simulink model "shabishiyan"  (R2021b)
settings: Solver=ode1  StartTime=0  StopTime=inf  FixedStep=0.005  RelTol=1e-3  EnableMultiTasking=on
libraries: gtbox x7, simulink x2
settings Model: SimulationMode=external  Creator=Administrator  LastModifiedBy=admin
settings SolverCC: AlgebraicLoopSolver=TrustRegion  AutoInsertRateTranBlk=on
settings DataIOCC: LimitDataPoints=on  SaveFormat=Array  ReturnWorkspaceOutputs=off
settings OptimizationCC: ExpressionDepthLimit=2147483647
settings DebuggingCC: UnderspecifiedInitializationDetection=Classic  MergeDetectMultiDrivingBlocksExec=none  SolverPrmCheckMsg=warning  MultiTaskRateTransMsg=warning  StateNameClashWarn=warning  SFUnexpectedBacktrackingDiag=warning  SFNoUnconditionalDefaultTransitionDiag=warning  SFExecutionAtInitializationDiag=none  SFMachineParentedDataDiag=warning  ArithmeticOperatorsInVariantConditions=warning
settings ModelReferenceCC: PropagateSignalLabelsOutOfModel=off
settings SFSimCC: SimUseLocalCustomCode=off  CustomCodeUndefinedFunction=UseInterfaceOnly
settings RTWCC: Description=Simulink Desktop Real-Time  SystemTargetFile=sldrt.tlc  TemplateMakefile=sldrt.tmf  RTWUseLocalCustomCode=off  RTWCompilerOptimization=on
settings CodeAppCC: MaxIdLength=95  StateflowObjectComments=on
settings SimulinkDesktopRealTimeCC: TargetPreCompLibLocation=C:\Program Files\MATLAB\R2021b\toolbox\sldrt\lib\win64  TargetLangStandard=C89/C90 (ANSI)  SupportVariableSizeSignals=off
settings ConfigComp: CovMetricSettings=dw  CovSaveCumulativeToWorkspaceVar=on  CovSaveSingleToWorkspaceVar=on  CovExternalEMLEnable=off

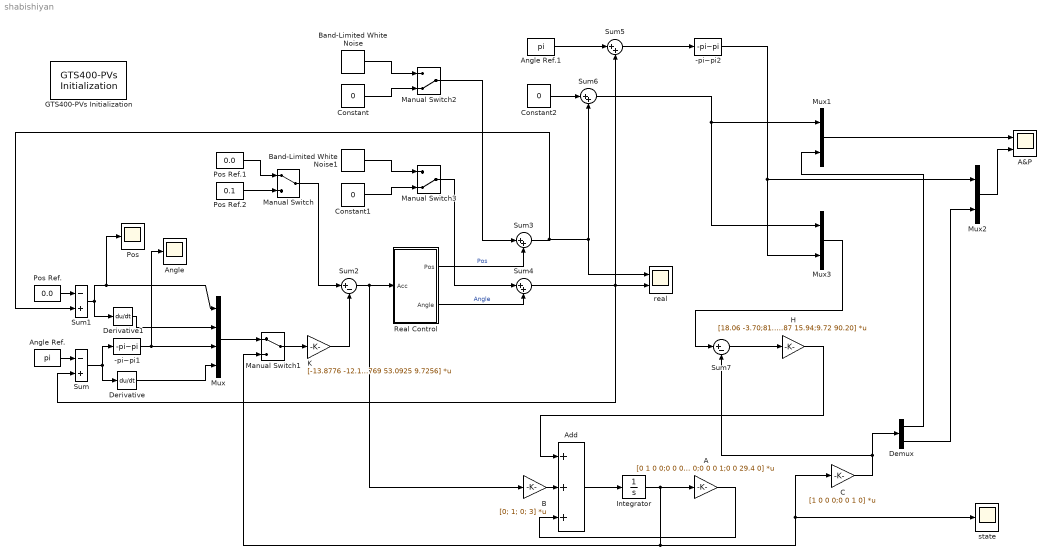
== system shabishiyan ==
  " -pi~pi1" : gtbox/GT-400-SV Function Blocks/ -pi~pi  Priority=1
      settings: SourceProductName=Googol Education Products v2.0
  " -pi~pi2" : gtbox/GT-400-SV Function Blocks/ -pi~pi  Priority=1
      settings: SourceProductName=Googol Education Products v2.0
  A : Gain  Gain=[0 1 0 0;0 0 0 0;0 0 0 1;0 0 29.4 0]  Multiplication=Matrix(K*u)
  A&P : Scope  NumInputPorts=2
  Add : Sum  Inputs=+++
  Angle : Scope
  Angle Ref. : Constant  Value=pi
  Angle Ref.1 : Constant  Value=pi
  B : Gain  Gain=[0; 1; 0; 3]  Multiplication=Matrix(K*u)
  Band-Limited White Noise : simulink/Sources/Band-Limited White Noise  Cov=[0.00001]  Ts=0.1  seed=[23341]
  Band-Limited White Noise1 : simulink/Sources/Band-Limited White Noise  Cov=[0.00001]  Ts=0.1  seed=[23341]
  C : Gain  Gain=[1 0 0 0;0 0 1 0]  Multiplication=Matrix(K*u)
  Constant : Constant  Value=0
  Constant1 : Constant  Value=0
  Constant2 : Constant  Value=0
  Demux : Demux  Outputs=2
  Derivative : Derivative
  Derivative1 : Derivative
  GTS400-PVs Initialization : gtbox/GTS-400-PV Function Blocks/GTS400-PVs Initialization  Priority=0  open=0  mode=0  servo=[1 0 0 0]  aft=[0 0 0 0]  pid1=[4.5 0 10]  pid2=[1 0 0]  pid3=[1 0 0]  pid4=[1 0 0]  enc1=on  enc2=on  enc3=on  enc4=on  lmt1=off  lmt2=off  lmt3=off  lmt4=off  cdno=1
      settings: SourceProductName=Googol Education Products v2.0
  H : Gain  Gain=[18.06 -3.70;81.37 -29.22;1.87 15.94;9.72 90.20]  Multiplication=Matrix(K*u)
  Integrator : Integrator
  K : Gain  Gain=[-13.8776 -12.1769 53.0925 9.7256]  Multiplication=Matrix(K*u)
  Manual Switch : ManualSwitch
  Manual Switch1 : ManualSwitch
  Manual Switch2 : ManualSwitch  CurrentSetting=0
  Manual Switch3 : ManualSwitch  CurrentSetting=0
  Mux : Mux
  Mux1 : Mux  Inputs=2
  Mux2 : Mux  Inputs=2
  Mux3 : Mux  Inputs=2
  Pos : Scope
  Pos Ref. : Constant  Value=0.0
  Pos Ref.1 : Constant  Value=0.0
  Pos Ref.2 : Constant  Value=0.1
  Real Control : Subsystem
  Sum : Sum  Inputs=-+  SaturateOnIntegerOverflow=on
  Sum1 : Sum  Inputs=-+  SaturateOnIntegerOverflow=on
  Sum2 : Sum  Inputs=|+-
  Sum{3..6} (4 alike) : Sum  Inputs=|++
  Sum7 : Sum  Inputs=|+-
  real : Scope  NumInputPorts=2
  state : Scope
  wires:
  Mux/1 -> Manual Switch1/1
  Sum/1 -> " -pi~pi1"/1, Derivative/1
  Derivative1/1 -> Mux/2
  Sum4/1 -> Sum5/2, real/2, Sum/2
  Derivative/1 -> Mux/4
  Sum3/1 -> real/1, Sum6/2, Sum1/2
  Pos Ref./1 -> Sum1/1
  Angle Ref./1 -> Sum/1
  " -pi~pi1"/1 -> Mux/3, Angle/1
  Sum1/1 -> Derivative1/1, Mux/1, Pos/1
  Pos Ref.1/1 -> Manual Switch/1
  Pos Ref.2/1 -> Manual Switch/2
  Manual Switch1/1 -> K/1
  Manual Switch/1 -> Sum2/1
  K/1 -> Sum2/2
  Band-Limited White Noise/1 -> Manual Switch2/1
  Constant/1 -> Manual Switch2/2
  Constant1/1 -> Manual Switch3/2
  Band-Limited White Noise1/1 -> Manual Switch3/1
  Manual Switch2/1 -> Sum3/1
  Real Control/1(Pos) -> Sum3/2  "Pos"
  Manual Switch3/1 -> Sum4/1
  Real Control/2(Angle) -> Sum4/2  "Angle"
  Constant2/1 -> Sum6/1
  Angle Ref.1/1 -> Sum5/1
  Sum5/1 -> " -pi~pi2"/1
  Sum6/1 -> Mux3/1, Mux1/1
  " -pi~pi2"/1 -> Mux3/2, Mux2/1
  Mux1/1 -> A&P/1
  Mux2/1 -> A&P/2
  Add/1 -> Integrator/1
  Mux3/1 -> Sum7/1
  Sum7/1 -> H/1
  H/1 -> Add/1
  B/1 -> Add/2
  Sum2/1 -> Real Control/1(Acc), B/1
  Integrator/1 -> C/1, state/1, Manual Switch1/2, A/1
  A/1 -> Add/3
  C/1 -> Demux/1, Sum7/2
  Demux/1 -> Mux1/2
  Demux/2 -> Mux2/2

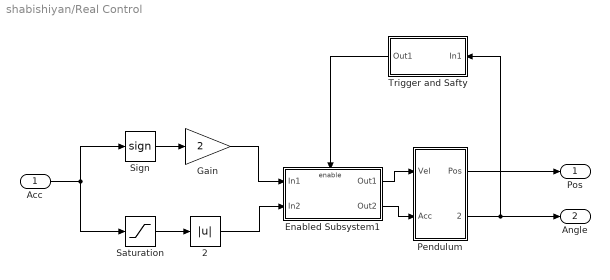
== system shabishiyan/Real Control ==
  Acc : Inport
  " 2" : Abs  SaturateOnIntegerOverflow=on
  Enabled Subsystem1 : Subsystem  TreatAsAtomicUnit=on
  Gain : Gain  Gain=2  SaturateOnIntegerOverflow=on  OutDataTypeStr=Inherit: Same as input  ParamDataTypeStr=Inherit: Same as input
  Pendulum : Subsystem
  Saturation : Saturate  UpperLimit=50  LowerLimit=-50
  Sign : Signum
  Trigger and Safty : Subsystem
  Pos : Outport
  Angle : Outport  Port=2
  wires:
  " 2"/1 -> Enabled Subsystem1/2(In2)
  Gain/1 -> Enabled Subsystem1/1(In1)
  Saturation/1 -> " 2"/1
  Pendulum/1(Pos) -> Pos/1
  Pendulum/2(Angle) -> Angle/1, Trigger and Safty/1(In1)
  Sign/1 -> Gain/1
  Acc/1 -> Sign/1, Saturation/1
  Trigger and Safty/1(Out1) -> Enabled Subsystem1/Enable
  Enabled Subsystem1/1(Out1) -> Pendulum/1(Vel)
  Enabled Subsystem1/2(Out2) -> Pendulum/2(Acc)

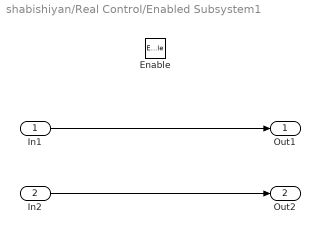
== system shabishiyan/Real Control/Enabled Subsystem1 ==
  In1 : Inport
  In2 : Inport  Port=2
  Enable : EnablePort
  Out1 : Outport
  Out2 : Outport  Port=2
  wires:
  In2/1 -> Out2/1
  In1/1 -> Out1/1

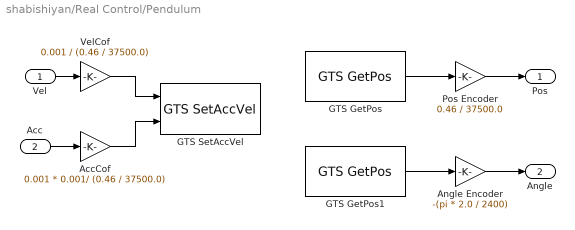
== system shabishiyan/Real Control/Pendulum ==
  Vel : Inport
  Acc : Inport  Port=2
  AccCof : Gain  Gain=0.001 * 0.001/ (0.46 / 37500.0)  SaturateOnIntegerOverflow=on  OutDataTypeStr=Inherit: Same as input  ParamDataTypeStr=Inherit: Same as input
  Angle Encoder : Gain  Gain=-(pi * 2.0 / 2400)  SaturateOnIntegerOverflow=on  OutDataTypeStr=Inherit: Same as input  ParamDataTypeStr=Inherit: Same as input
  GTS GetPos : gtbox/GTS-400-PV Function Blocks/GTS GetPos  Priority=1  axis=1
      settings: SourceProductName=Googol Education Products v2.0
  GTS GetPos1 : gtbox/GTS-400-PV Function Blocks/GTS GetPos  Priority=1  axis=2
      settings: SourceProductName=Googol Education Products v2.0
  GTS SetAccVel : gtbox/GTS-400-PV Function Blocks/GTS SetAccVel  Priority=1  Axis=1  vel=0.1  pos=50000  limit=0
      settings: SourceProductName=Googol Education Products v2.0
  Pos Encoder : Gain  Gain=0.46 / 37500.0  SaturateOnIntegerOverflow=on  OutDataTypeStr=Inherit: Same as input  ParamDataTypeStr=Inherit: Same as input
  VelCof : Gain  Gain=0.001 / (0.46 / 37500.0)  SaturateOnIntegerOverflow=on  OutDataTypeStr=Inherit: Same as input  ParamDataTypeStr=Inherit: Same as input
  Pos : Outport
  Angle : Outport  Port=2
  wires:
  Angle Encoder/1 -> Angle/1
  Pos Encoder/1 -> Pos/1
  GTS GetPos1/1 -> Angle Encoder/1
  Acc/1 -> AccCof/1
  Vel/1 -> VelCof/1
  GTS GetPos/1 -> Pos Encoder/1
  AccCof/1 -> GTS SetAccVel/2
  VelCof/1 -> GTS SetAccVel/1

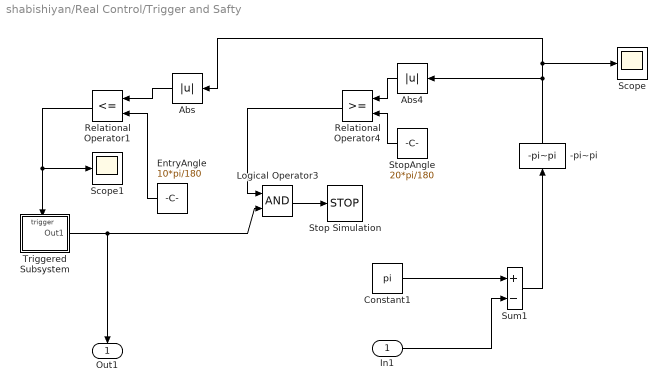
== system shabishiyan/Real Control/Trigger and Safty ==
  In1 : Inport
  " -pi~pi" : gtbox/GT-400-SV Function Blocks/ -pi~pi
      settings: SourceProductName=Googol Education Products v2.0
  Abs : Abs  SaturateOnIntegerOverflow=on
  Abs4 : Abs  SaturateOnIntegerOverflow=on
  Constant1 : Constant  Value=pi
  EntryAngle : Constant  Value=10*pi/180
  Logical Operator3 : Logic  AllPortsSameDT=off
  Relational Operator1 : RelationalOperator  Operator=<=  RndMeth=Nearest
  Relational Operator4 : RelationalOperator  RndMeth=Nearest
  Scope : Scope
  Scope1 : Scope
  Stop Simulation : Stop
  StopAngle : Constant  Value=20*pi/180
  Sum1 : Sum  Inputs=+-  SaturateOnIntegerOverflow=on
  Triggered Subsystem : Subsystem  TreatAsAtomicUnit=on
  Out1 : Outport
  wires:
  Relational Operator4/1 -> Logical Operator3/1
  StopAngle/1 -> Relational Operator4/2
  Abs4/1 -> Relational Operator4/1
  Abs/1 -> Relational Operator1/1
  EntryAngle/1 -> Relational Operator1/2
  Relational Operator1/1 -> Scope1/1, Triggered Subsystem/Trigger
  Triggered Subsystem/1(Out1) -> Logical Operator3/2, Out1/1
  Logical Operator3/1 -> Stop Simulation/1
  " -pi~pi"/1 -> Abs4/1, Scope/1, Abs/1
  Constant1/1 -> Sum1/1
  In1/1 -> Sum1/2
  Sum1/1 -> " -pi~pi"/1

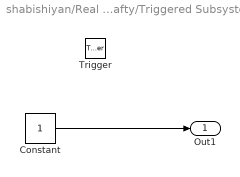
== system shabishiyan/Real Control/Trigger and Safty/Triggered Subsystem ==
  Trigger : TriggerPort  VariantControl=(inherit)
  Constant : Constant
  Out1 : Outport  InitialOutput=0
  wires:
  Constant/1 -> Out1/1
